simulink model "VehicleDynamics_Module"  (R2025a)
settings: Solver=VariableStepAuto
undefined symbols (not defined in the file): a_brake_mps2, a_throttle_mps2
settings Model: Creator=ASUS  LastModifiedBy=ASUS

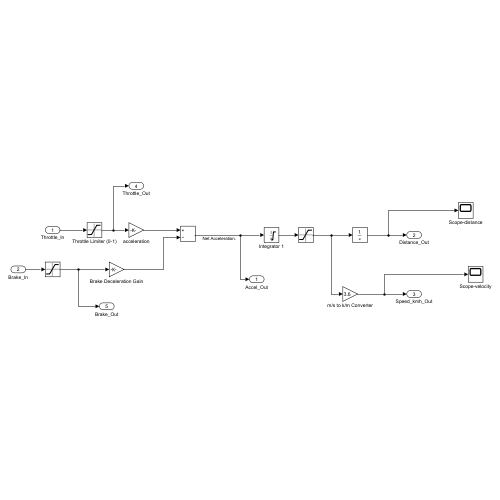
[thumbnail: Simulink's stored preview of the top-level diagram]
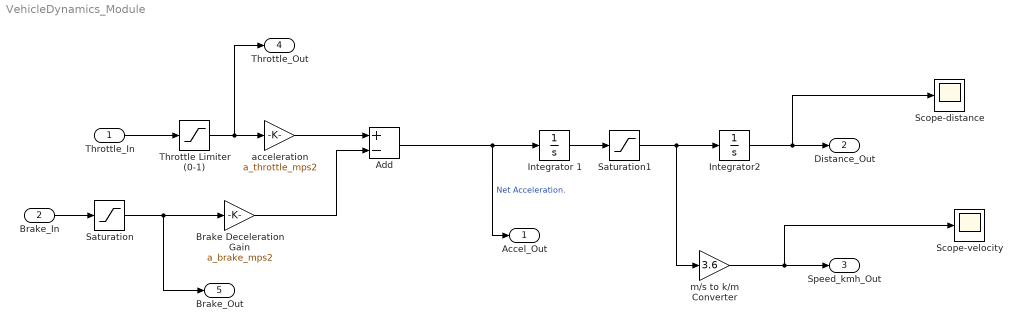
== system VehicleDynamics_Module ==
  Throttle_In : Inport
  Brake_In : Inport  Port=2
  Add : Sum  Inputs=+-
  Brake Deceleration Gain : Gain  Gain=a_brake_mps2
  Integrator 1 : Integrator  LimitOutput=on  UpperSaturationLimit=36
  Integrator2 : Integrator
  Saturation : Saturate  UpperLimit=1  LowerLimit=0
  Saturation1 : Saturate  UpperLimit=inf  LowerLimit=0
  Scope-distance : Scope
      settings: ActiveDisplayYMinimum=-150.44969096704656  ActiveDisplayYMaximum=110.52038836645281
  Scope-velocity : Scope
      settings: ActiveDisplayYMinimum=-16.651487801579165  ActiveDisplayYMaximum=120.5928135374248
  Throttle Limiter (0-1) : Saturate  UpperLimit=1  LowerLimit=0
  acceleration : Gain  Gain=a_throttle_mps2
  m/s to k/m Converter : Gain  Gain=3.6
  Accel_Out : Outport
  Distance_Out : Outport  Port=2
  Speed_kmh_Out : Outport  Port=3
  Throttle_Out : Outport  Port=4
  Brake_Out : Outport  Port=5
  wires:
  Integrator2/1 -> Scope-distance/1, Distance_Out/1
  m/s to k/m Converter/1 -> Scope-velocity/1, Speed_kmh_Out/1
  Throttle_In/1 -> Throttle Limiter (0-1)/1
  Brake_In/1 -> Saturation/1
  Saturation/1 -> Brake_Out/1, Brake Deceleration Gain/1
  Brake Deceleration Gain/1 -> Add/2
  acceleration/1 -> Add/1
  Add/1 -> Accel_Out/1, Integrator 1/1  "Net Acceleration."
  Integrator 1/1 -> Saturation1/1
  Saturation1/1 -> m/s to k/m Converter/1, Integrator2/1
  Throttle Limiter (0-1)/1 -> Throttle_Out/1, acceleration/1
